simulink model "Hardware_deploy_model"  (R2019a)
settings: Solver=FixedStepDiscrete  StartTime=0.0  StopTime=inf  RelTol=1e-3
model workspace (MAT data in the model file):
  actuatorCentres.aileron.left = 0
  actuatorCentres.aileron.right = 0
  actuatorCentres.elevator.right = 0
  actuatorCentres.elevator.left = 0
  actuatorCentres.flap.left = 0
  actuatorCentres.flap.right = 0
  actuatorCentres.rudder = 0
  loggingSampleTime = Simulink.Parameter
  loggingSampleTime.Value = 1
  loggingSampleTime.DataType = 'double'
  loggingSampleTime.Dimensions = [1 1]
  sensorSampleTime = Simulink.Parameter
  sensorSampleTime.Value = 0.01
  sensorSampleTime.DataType = 'double'
  sensorSampleTime.Dimensions = [1 1]
  servoPins.aileron.left = 9
  servoPins.aileron.right = 10
  servoPins.elevator.left = 7
  servoPins.elevator.right = 8
  servoPins.rudder = 11
  servoPins.flap.left = 5
  servoPins.flap.right = 6
undefined symbols (not defined in the file or in its folder): Aileron, deflectionLimits, DiscIntNeverNeededParam, Discrete, Elevator, Newton, Raphson, Time
libraries: simulink x13, arduinolib x6, ctrlSharedLib x3, aerolibtransform2 x3, sharedtransform x2, aerolibutil x1, simulink_extras x1
settings Model: ExtModeTrigDuration=2  Creator=Aliak  LastModifiedBy=Aliak
settings OptimizationCC: DefaultParameterBehavior=Inlined  GainParamInheritBuiltInType=on  UseFloatMulNetSlope=on  DefaultUnderspecifiedDataType=single  UseSpecifiedMinMax=on  InlineInvariantSignals=on  BitfieldContainerType=uchar_T  MemcpyThreshold=32  PassReuseOutputArgsAs=Individual arguments  ActiveStateOutputEnumStorageType=Smallest  ZeroExternalMemoryAtStartup=off  ZeroInternalMemoryAtStartup=off  NoFixptDivByZeroProtection=on  EfficientFloat2IntCast=on  EfficientMapNaN2IntZero=off  LifeSpan=0.02  MaxStackSize=inf  SimCompilerOptimization=on  OptimizeBlockOrder=speed  DifferentSizesBufferReuse=on
settings DebuggingCC: WriteAfterWriteMsg=EnableAllAsError  AlgebraicLoopMsg=error  IntegerOverflowMsg=error  ParameterUnderflowMsg=error  ParameterPrecisionLossMsg=none  ParameterTunabilityLossMsg=error  AllowSymbolicDim=off  ModelReferenceIOMsg=error  StrictBusMsg=ErrorOnBusTreatedAsVector  NonBusSignalsTreatedAsBus=error  SFInvalidInputDataAccessInChartInitDiag=error  SFTransitionOutsideNaturalParentDiag=error  SFUnreachableExecutionPathDiag=error  SFUndirectedBroadcastEventsDiag=error  SFTransitionActionBeforeConditionDiag=error  IntegerSaturationMsg=error
settings HardwareCC: ProdBitPerInt=16  ProdBitPerPointer=16  ProdBitPerSizeT=16  ProdBitPerPtrDiffT=16  ProdLargestAtomicFloat=None  ProdWordSize=8  ProdLongLongMode=on  ProdHWDeviceType=Atmel->AVR
settings ModelReferenceCC: EnableParallelModelReferenceBuilds=on  ModelReferenceNumInstancesAllowed=Single  ModelReferenceMinAlgLoopOccurrences=on
settings SFSimCC: SimParseCustomCode=off  MATLABDynamicMemAlloc=off
settings RTWCC: SystemTargetFile=ert.tlc  HardwareBoard=Arduino Mega 2560  TemplateMakefile=ert_default_tmf  Toolchain=Arduino AVR  BuildConfiguration=Faster Runs  IncludeHyperlinkInReport=on  CheckMdlBeforeBuild=Warning
settings CodeAppCC: ForceParamTrailComments=on  IgnoreCustomStorageClasses=off  IgnoreTestpoints=on  OperatorAnnotations=on  SimulinkDataObjDesc=on  SFDataObjDesc=on  MATLABFcnDesc=on  InsertBlockDesc=on
settings ERTTargetCC: UtilityFuncGeneration=Shared location  DynamicStringBufferSize=128  IncludeMdlTerminateFcn=off  CombineSignalStateStructs=on  SuppressErrorStatus=on  SupportAbsoluteTime=off  SupportComplex=off  PreserveIfCondition=on
settings ConfigComp: CovScope=ReferencedModels

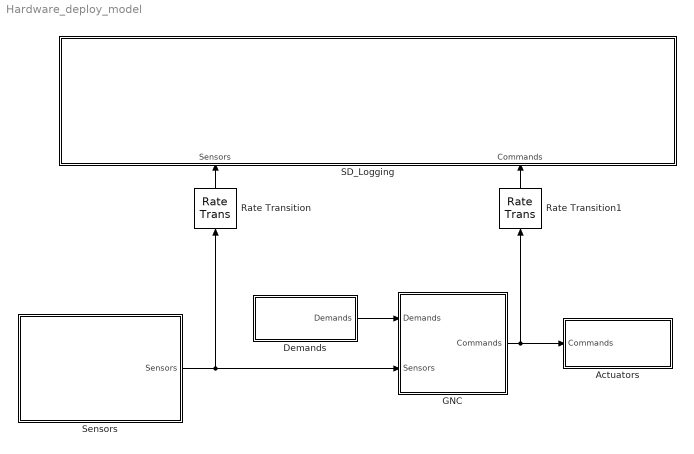
== system Hardware_deploy_model ==
  Actuators : Subsystem  VariantControl=SimType == 1
  Demands : Subsystem
  GNC : Subsystem  VariantControl=SimType==1
  Rate Transition : RateTransition  Deterministic=off  OutPortSampleTime=0.2
  Rate Transition1 : RateTransition  Deterministic=off  OutPortSampleTime=0.2
  SD_Logging : Subsystem  VariantControl=SecArd == 1
  Sensors : Subsystem  VariantControl=SimType==1
  wires:
  Sensors/1(" Sensors") -> GNC/2(Sensors), Rate Transition/1
  GNC/1(Commands) -> Rate Transition1/1, Actuators/1(Commands)
  Rate Transition/1 -> SD_Logging/1("Sensors ")
  Demands/1(Demands) -> GNC/1(Demands)
  Rate Transition1/1 -> SD_Logging/2(Commands)

== system Hardware_deploy_model/Actuators ==
  Commands : Inport  OutDataTypeStr=Bus: Commands
  Aileron Servos : arduinolib/Standard Servo Write  pinNumber=6  ServoIndex=0  blockPlatform=ARDUINO
      settings: SourceProductName=Simulink Support Package for Arduino Hardware
  Bus Selector : BusSelector  OutputSignals=Aileron,Elevator
  Constant : Constant  Value=actuatorCentres.aileron.left  VectorParams1D=off
  Constant1 : Constant  Value=actuatorCentres.elevator.left  VectorParams1D=off
  Elevator Servo : arduinolib/Standard Servo Write  pinNumber=5  ServoIndex=1  blockPlatform=ARDUINO
      settings: SourceProductName=Simulink Support Package for Arduino Hardware
  Initialize Function : Subsystem  Commented=on  TreatAsAtomicUnit=on
  Saturation : Saturate  Commented=through  UpperLimit=deflectionLimits.aileron.max  LowerLimit=deflectionLimits.aileron.min
  Saturation1 : Saturate  Commented=through  UpperLimit=deflectionLimits.elevator.max  LowerLimit=deflectionLimits.elevator.min
  Subtract : Sum  Inputs=-+  RndMeth=Simplest
  Subtract1 : Sum  Inputs=-+
  wires:
  Commands/1 -> Bus Selector/1
  Saturation1/1 -> Subtract1/2
  Bus Selector/2 -> Saturation1/1  "<Elevator>"
  Subtract1/1 -> Elevator Servo/1
  Constant1/1 -> Subtract1/1
  Bus Selector/1 -> Saturation/1  "<Aileron>"
  Saturation/1 -> Subtract/2
  Constant/1 -> Subtract/1
  Subtract/1 -> Aileron Servos/1

== system Hardware_deploy_model/Demands ==
  Bus Creator : BusCreator  Inputs=2  OutDataTypeStr=Bus: Demands
  Constant : Constant  Value=90  VectorParams1D=off  OutDataTypeStr=single
  Constant1 : Constant  Value=60  VectorParams1D=off  OutDataTypeStr=single
  Demands : Outport
  wires:
  Constant/1 -> Bus Creator/1  "Heading"
  Constant1/1 -> Bus Creator/2  "Altitude"
  Bus Creator/1 -> Demands/1

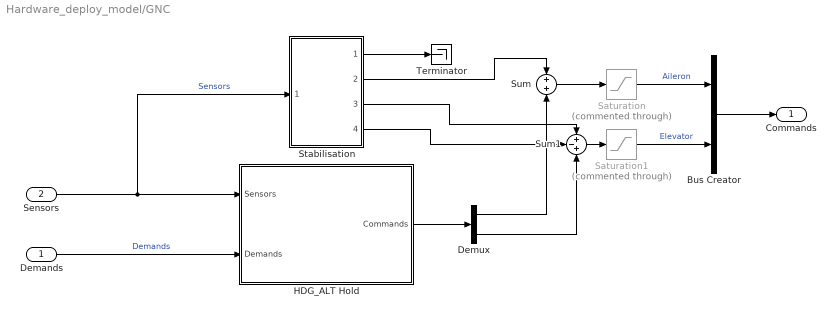
== system Hardware_deploy_model/GNC ==
  Demands : Inport  OutDataTypeStr=Bus: Demands
  Sensors : Inport  Port=2  OutDataTypeStr=Bus: Sensors
  Bus Creator : BusCreator  Inputs=Aileron,Elevator  OutDataTypeStr=Bus: Commands
  Demux : Demux  Outputs=2
  HDG_ALT Hold : Subsystem
  Saturation : Saturate  Commented=through  UpperLimit=deflectionLimits.aileron.max  LowerLimit=deflectionLimits.aileron.min
  Saturation1 : Saturate  Commented=through  UpperLimit=deflectionLimits.elevator.max  LowerLimit=deflectionLimits.elevator.min
  Stabilisation : Subsystem
  Sum : Sum
  Sum1 : Sum  Inputs=+-+
  Terminator : Terminator
  Commands : Outport
  wires:
  Bus Creator/1 -> Commands/1
  Sum/1 -> Saturation/1
  Sum1/1 -> Saturation1/1
  HDG_ALT Hold/1(Commands) -> Demux/1
  Demux/1 -> Sum/2
  Sensors/1 -> Stabilisation/1(Sensors), HDG_ALT Hold/1(Sensors)  "Sensors"
  Demands/1 -> HDG_ALT Hold/2(Demands)  "Demands"
  Demux/2 -> Sum1/3
  Stabilisation/2(Roll Stab) -> Sum/1
  Stabilisation/3(Pitch Stab) -> Sum1/1
  Stabilisation/1(Yaw Stab) -> Terminator/1
  Stabilisation/4(Stall Stab) -> Sum1/2
  Saturation/1 -> Bus Creator/1  "Aileron"
  Saturation1/1 -> Bus Creator/2  "Elevator"

== system Hardware_deploy_model/SD_Logging ==
  "Sensors " : Inport  OutDataTypeStr=Bus: Sensors
  Commands : Inport  Port=2  OutDataTypeStr=Bus: Commands
  Bus Selector : BusSelector  OutputSignals=X_e,V_e,phi_theta_psi,pqr
  Bus Selector1 : BusSelector  OutputSignals=Aileron,Elevator
  Demux{,1..3} (4 alike) : Demux  Outputs=3
  MATLAB System : MATLABSystem  System=SDLogger  SimulateUsing=Code generation
      mask Type: SDLogger
      mask Display:
      | disp('SDLogger');
      | port_label('input',1,'data');
  Mux : Mux  Inputs=14
  wires:
  "Sensors "/1 -> Bus Selector/1
  Bus Selector/1 -> Demux/1  "<X_e>"
  Bus Selector/3 -> Demux1/1  "<phi_theta_psi>"
  Bus Selector/4 -> Demux2/1  "<pqr>"
  Bus Selector/2 -> Demux3/1  "<V_e>"
  Demux/1 -> Mux/1
  Demux/2 -> Mux/2
  Demux/3 -> Mux/3
  Demux3/1 -> Mux/4
  Demux3/2 -> Mux/5
  Demux3/3 -> Mux/6
  Demux1/1 -> Mux/7
  Demux1/2 -> Mux/8
  Demux1/3 -> Mux/9
  Demux2/1 -> Mux/10
  Demux2/2 -> Mux/11
  Demux2/3 -> Mux/12
  Mux/1 -> MATLAB System/1
  Commands/1 -> Bus Selector1/1
  Bus Selector1/1 -> Mux/13  "<Aileron>"
  Bus Selector1/2 -> Mux/14  "<Elevator>"

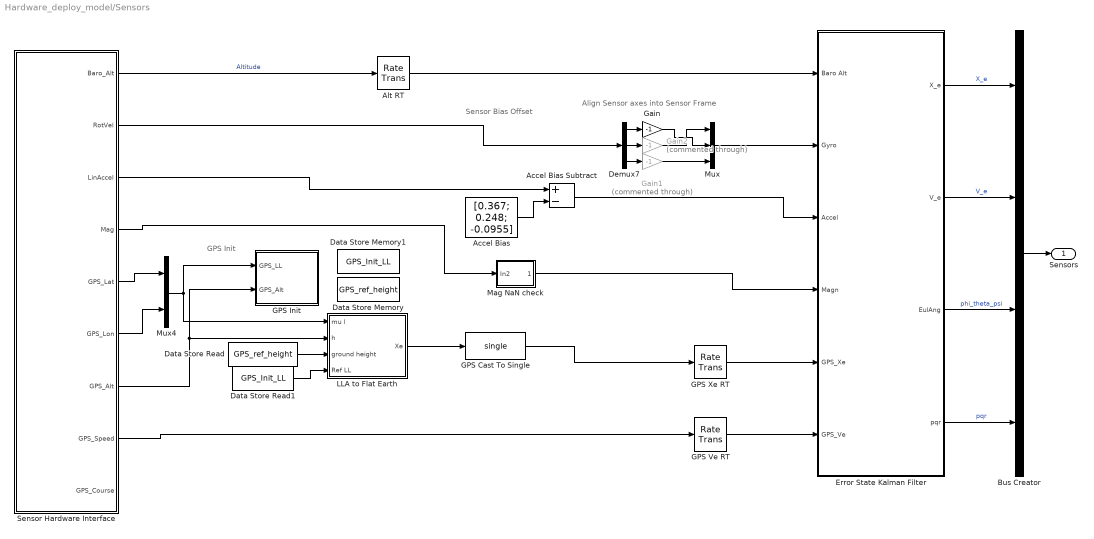
== system Hardware_deploy_model/Sensors ==
  note: GPS Init
  note: Sensor Bias Offset
  note: Align Sensor axes into Sensor Frame
  Accel Bias : Constant  Value=[0.367; 0.248; -0.0955]  VectorParams1D=off
  Accel Bias Subtract : Sum  Inputs=+-  OutDataTypeStr=single
  Alt RT : RateTransition  Deterministic=off
  Bus Creator : BusCreator  Inputs=4  OutDataTypeStr=Bus: Sensors
      settings: InheritFromInputs=off
  Data Store Memory : DataStoreMemory  DataStoreName=GPS_ref_height  ReadBeforeWriteMsg=warning  WriteAfterWriteMsg=warning  WriteAfterReadMsg=warning  ShowAdditionalParam=off  OutDataTypeStr=single
  Data Store Memory1 : DataStoreMemory  DataStoreName=GPS_Init_LL  ReadBeforeWriteMsg=warning  WriteAfterWriteMsg=warning  WriteAfterReadMsg=warning  InitialValue=[0 0]  ShowAdditionalParam=off  OutDataTypeStr=single
  Data Store Read : DataStoreRead  DataStoreName=GPS_ref_height  DataStoreElements=GPS_ref_height
  Data Store Read1 : DataStoreRead  DataStoreName=GPS_Init_LL
  Demux7 : Demux  Outputs=3
  Error State Kalman Filter : Subsystem
  GPS Cast To Single : DataTypeConversion  OutDataTypeStr=single  RndMeth=Simplest
  GPS Init : Subsystem
  GPS Ve RT : RateTransition  Deterministic=off
  GPS Xe RT : RateTransition  Deterministic=off
  Gain : Gain  Gain=-1
  Gain1 : Gain  Commented=through  Gain=-1
  Gain2 : Gain  Commented=through  Gain=-1
  LLA to Flat Earth : Subsystem
  Mag NaN check : Subsystem
  Mux : Mux  Inputs=3
  Mux4 : Mux  Inputs=2
  Sensor Hardware Interface : Subsystem  VariantControl=SimType==1
  " Sensors" : Outport
  wires:
  Error State Kalman Filter/3(EulAng) -> Bus Creator/3  "phi_theta_psi"
  Error State Kalman Filter/2(V_e) -> Bus Creator/2  "V_e"
  Error State Kalman Filter/1(X_e) -> Bus Creator/1  "X_e"
  Error State Kalman Filter/4(pqr) -> Bus Creator/4  "pqr"
  Bus Creator/1 -> " Sensors"/1
  GPS Ve RT/1 -> Error State Kalman Filter/6(GPS_Ve)
  GPS Cast To Single/1 -> GPS Xe RT/1
  Sensor Hardware Interface/1(Baro_Alt) -> Alt RT/1  "Altitude"
  Sensor Hardware Interface/4(Mag) -> Mag NaN check/1(In2)
  Demux7/3 -> Gain1/1
  Sensor Hardware Interface/7(GPS_Alt) -> LLA to Flat Earth/2(h), GPS Init/2(GPS_Alt)
  Sensor Hardware Interface/5(GPS_Lat) -> Mux4/1
  Data Store Read1/1 -> LLA to Flat Earth/4(Ref LL)
  Sensor Hardware Interface/8(GPS_Speed) -> GPS Ve RT/1
  Sensor Hardware Interface/6(GPS_Lon) -> Mux4/2
  LLA to Flat Earth/1(Xe) -> GPS Cast To Single/1
  Gain1/1 -> Mux/3
  Demux7/1 -> Gain/1
  Mag NaN check/1(Out1) -> Error State Kalman Filter/4(Magn)
  Accel Bias Subtract/1 -> Error State Kalman Filter/3(Accel)
  Mux/1 -> Error State Kalman Filter/2(Gyro)
  Sensor Hardware Interface/2(RotVel) -> Demux7/1
  Alt RT/1 -> Error State Kalman Filter/1(Baro Alt)
  Gain/1 -> Mux/2
  Sensor Hardware Interface/3(LinAccel) -> Accel Bias Subtract/1
  Data Store Read/1 -> LLA to Flat Earth/3(ground height)
  GPS Xe RT/1 -> Error State Kalman Filter/5(GPS_Xe)
  Mux4/1 -> LLA to Flat Earth/1(mu l), GPS Init/1(GPS_LL)
  Gain2/1 -> Mux/1
  Accel Bias/1 -> Accel Bias Subtract/2
  Demux7/2 -> Gain2/1

== system Hardware_deploy_model/Actuators/Initialize Function ==
  Aileron Servos : arduinolib/Standard Servo Write  pinNumber=servoPins.aileron.right  ServoIndex=0  blockPlatform=ARDUINO
      settings: SourceProductName=Simulink Support Package for Arduino Hardware
  Elevator Servo : arduinolib/Standard Servo Write  pinNumber=servoPins.elevator.right  ServoIndex=0  blockPlatform=ARDUINO
      settings: SourceProductName=Simulink Support Package for Arduino Hardware
  Event Listener : EventListener  DisableCoverage=on  EventName=reset
  Flap Servo : arduinolib/Standard Servo Write  pinNumber=servoPins.flap.right  ServoIndex=0  blockPlatform=ARDUINO
      settings: SourceProductName=Simulink Support Package for Arduino Hardware
  Rudder Servo : arduinolib/Standard Servo Write  pinNumber=servoPins.rudder  ServoIndex=0  blockPlatform=ARDUINO
      settings: SourceProductName=Simulink Support Package for Arduino Hardware
  Step : Step  After=180  SampleTime=0
  Step1 : Step  Time=6  After=180  SampleTime=0
  Sum : Sum  Inputs=+-
  wires:
  Sum/1 -> Flap Servo/1, Rudder Servo/1, Elevator Servo/1, Aileron Servos/1
  Step/1 -> Sum/1
  Step1/1 -> Sum/2

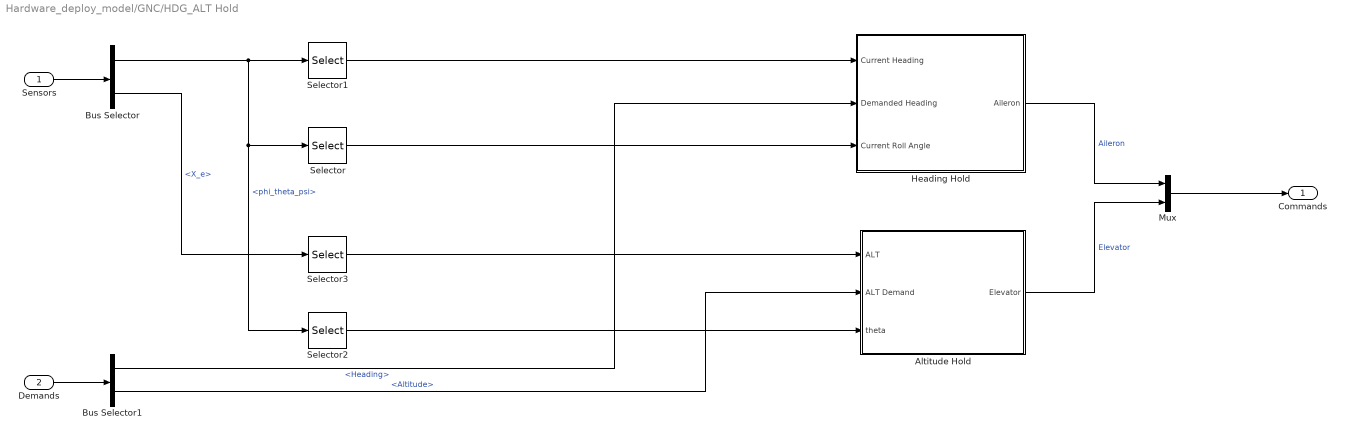
== system Hardware_deploy_model/GNC/HDG_ALT Hold ==
  Sensors : Inport  OutDataTypeStr=Bus: Sensors
  Demands : Inport  Port=2  OutDataTypeStr=Bus: Demands
  Altitude Hold : Subsystem
      settings: UndoDeleteFcn=Stateflow.SLINSF.SimulinkMan.restorePreDeleteFcn  PreDeleteFcn=Stateflow.SLINSF.SimulinkMan.removePreDeleteFcn
  Bus Selector : BusSelector  OutputSignals=phi_theta_psi,X_e
  Bus Selector1 : BusSelector  OutputSignals=Heading,Altitude
  Heading Hold : Subsystem
  Mux : Mux  Inputs=2
  Selector : Selector  IndexMode=Zero-based  InputPortWidth=3  IndexOptions=Index vector (dialog)  Indices=[0]  OutputSizes=1
  Selector1 : Selector  IndexMode=Zero-based  InputPortWidth=3  IndexOptions=Index vector (dialog)  Indices=[2]  OutputSizes=1
  Selector2 : Selector  IndexMode=Zero-based  InputPortWidth=3  IndexOptions=Index vector (dialog)  Indices=[1]  OutputSizes=1
  Selector3 : Selector  IndexMode=Zero-based  InputPortWidth=3  IndexOptions=Index vector (dialog)  Indices=[2]  OutputSizes=1
  Commands : Outport
  wires:
  Selector1/1 -> Heading Hold/1(Current Heading)
  Selector3/1 -> Altitude Hold/1(ALT)
  Bus Selector1/2 -> Altitude Hold/2(ALT Demand)  "<Altitude>"
  Bus Selector/1 -> Selector1/1, Selector/1, Selector2/1  "<phi_theta_psi>"
  Bus Selector1/1 -> Heading Hold/2(Demanded Heading)  "<Heading>"
  Bus Selector/2 -> Selector3/1  "<X_e>"
  Demands/1 -> Bus Selector1/1
  Selector/1 -> Heading Hold/3(Current Roll Angle)
  Sensors/1 -> Bus Selector/1
  Selector2/1 -> Altitude Hold/3(theta)
  Altitude Hold/1(Elevator) -> Mux/2  "Elevator"
  Mux/1 -> Commands/1
  Heading Hold/1(Aileron) -> Mux/1  "Aileron"

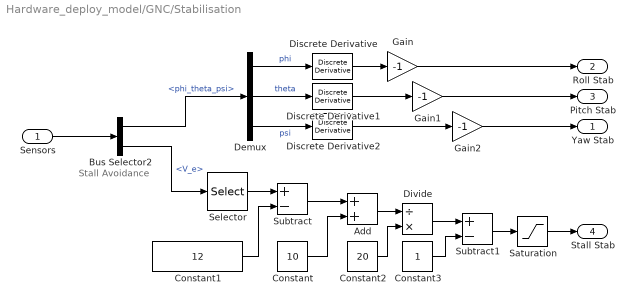
== system Hardware_deploy_model/GNC/Stabilisation ==
  note: Stall Avoidance
  Sensors : Inport
  Add : Sum
  Bus Selector2 : BusSelector  OutputSignals=phi_theta_psi,V_e
  Constant : Constant  Value=10  OutDataTypeStr=single
  Constant1 : Constant  Value=12  OutDataTypeStr=single
  Constant2 : Constant  Value=20  OutDataTypeStr=single
  Constant3 : Constant  OutDataTypeStr=single
  Demux : Demux  Outputs=3
  Discrete Derivative : simulink/Discrete/Discrete Derivative  gainval=1.0  ICPrevScaledInput=0.0  OutMin=-50  OutMax=50  OutDataType=fixdt(1, 16)  OutScaling=2^-10  RndMeth=Simplest  DoSatur=on
  Discrete Derivative1 : simulink/Discrete/Discrete Derivative  gainval=1.0  ICPrevScaledInput=0.0  OutMin=-50  OutMax=50  OutDataType=fixdt(1, 16)  OutScaling=2^-10  RndMeth=Simplest  DoSatur=on
  Discrete Derivative2 : simulink/Discrete/Discrete Derivative  gainval=1.0  ICPrevScaledInput=0.0  OutMin=-50  OutMax=50  OutDataType=fixdt(1, 16)  OutScaling=2^-10  RndMeth=Simplest  DoSatur=on
  Divide : Product  Inputs=/*
  Gain : Gain  Gain=-1
  Gain1 : Gain  Gain=-1
  Gain2 : Gain  Gain=-1
  Saturation : Saturate  UpperLimit=1  LowerLimit=0
  Selector : Selector  IndexMode=Zero-based  InputPortWidth=3  IndexOptions=Index vector (dialog)  Indices=[0]  OutputSizes=1
  Subtract : Sum  Inputs=+-
  Subtract1 : Sum  Inputs=+-
  Yaw Stab : Outport
  Roll Stab : Outport  Port=2
  Pitch Stab : Outport  Port=3
  Stall Stab : Outport  Port=4
  wires:
  Gain2/1 -> Yaw Stab/1
  Bus Selector2/2 -> Selector/1  "<V_e>"
  Discrete Derivative2/1 -> Gain2/1
  Selector/1 -> Subtract/1
  Sensors/1 -> Bus Selector2/1
  Demux/2 -> Discrete Derivative1/1  "theta"
  Demux/1 -> Discrete Derivative/1  "phi"
  Demux/3 -> Discrete Derivative2/1  "psi"
  Discrete Derivative1/1 -> Gain1/1
  Discrete Derivative/1 -> Gain/1
  Bus Selector2/1 -> Demux/1  "<phi_theta_psi>"
  Gain/1 -> Roll Stab/1
  Gain1/1 -> Pitch Stab/1
  Constant1/1 -> Subtract/2
  Saturation/1 -> Stall Stab/1
  Subtract/1 -> Add/1
  Constant/1 -> Add/2
  Add/1 -> Divide/1
  Constant2/1 -> Divide/2
  Divide/1 -> Subtract1/1
  Constant3/1 -> Subtract1/2
  Subtract1/1 -> Saturation/1

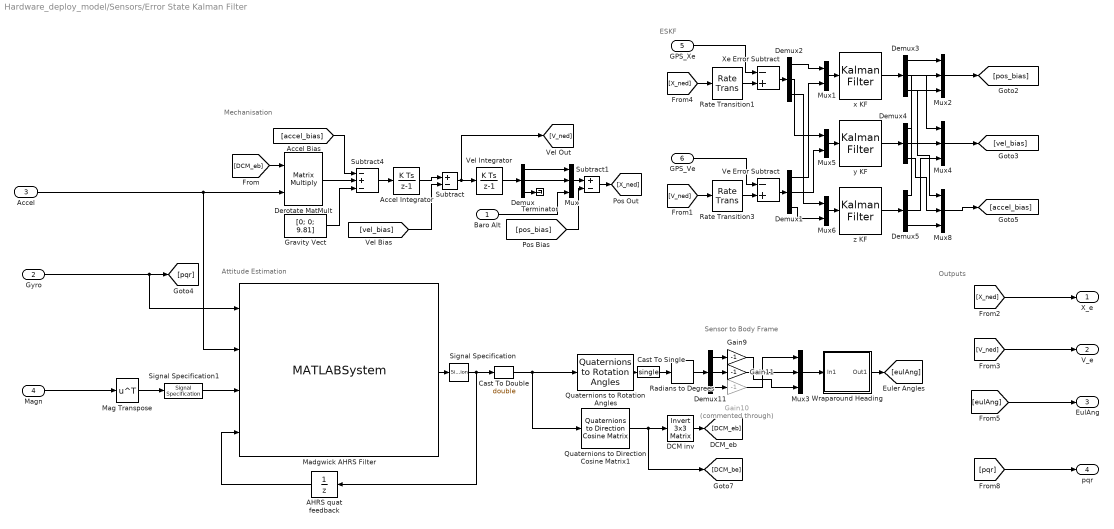
== system Hardware_deploy_model/Sensors/Error State Kalman Filter ==
  note: Attitude Estimation
  note: Mechanisation
  note: ESKF
  note: Outputs
  note: Sensor to Body Frame
  Baro Alt : Inport
  Gyro : Inport  Port=2
  Accel : Inport  Port=3
  Magn : Inport  Port=4
  GPS_Xe : Inport  Port=5
  GPS_Ve : Inport  Port=6
  AHRS quat feedback : UnitDelay  InitialCondition=[1 0 0 0]  SampleTime=sensorSampleTime  HasFrameUpgradeWarning=on
  Accel Integrator : DiscreteIntegrator  gainval=1  SampleTime=-1  ICPrevOutput=DiscIntNeverNeededParam  ICPrevScaledInput=DiscIntNeverNeededParam
  Cast To Double : DataTypeConversion  OutDataTypeStr=double
  Cast To Single : DataTypeConversion  OutDataTypeStr=single
  DCM inv : aerolibutil/Invert  3x3 Matrix
  Demux{,1..5,11} (7 alike) : Demux  Outputs=3
  Derotate MatMult : Product  Multiplication=Matrix(*)  OutDataTypeStr=single  RndMeth=Simplest
  Gain10 : Gain  Commented=through  Gain=-1
  Gain11 : Gain  Gain=-1
  Gain9 : Gain  Gain=-1
  Gravity Vect : Constant  Value=[0; 0; 9.81]  VectorParams1D=off  OutDataTypeStr=single
  Madgwick AHRS Filter : MATLABSystem  System=MadgwickAHRSFilter  SamplePeriod=sensorSampleTime  Beta=1  SimulateUsing=Code generation
      mask Type: MadgwickAHRSFilter
      mask Display:
      | disp('MadgwickAHRSFilter');
      | port_label('input',1,'Gyroscope');
      | port_label('input',2,'Accelerometer');
      | port_label('input',3,'Magnetometer');
      | port_label('input',4,'q');
      | port_label('output',1,'quat');
  Mag Transpose : Math  Operator=transpose  SaturateOnIntegerOverflow=on
  Mux{,2..4,8} (5 alike) : Mux  Inputs=3
  Mux1 : Mux  Inputs=2
  Mux5 : Mux  Inputs=2
  Mux6 : Mux  Inputs=2
  Quaternions to Direction Cosine Matrix1 : sharedtransform/Quaternions to  Direction Cosine Matrix  aMode=aMode
      settings: SourceProductName=Aerospace Blockset  SourceProductBaseCode=AE
  Quaternions to Rotation Angles : sharedtransform/Quaternions to Rotation Angles  rotationOrder=ZYX  aMode=aMode
      settings: SourceProductBaseCode=AE
  Radians to Degrees : simulink_extras/Transformations/Radians to Degrees
  Rate Transition1 : RateTransition  Deterministic=off  OutPortSampleTime=1
  Rate Transition3 : RateTransition  Deterministic=off  OutPortSampleTime=1
  Signal Specification : SignalSpecification  OutDataTypeStr=single  Dimensions=[1 4]
  Signal Specification1 : SignalSpecification  OutDataTypeStr=single  Dimensions=[1 3]
  Subtract : Sum  Inputs=+-
  Subtract1 : Sum  Inputs=+-
  Subtract4 : Sum  Inputs=-+-  AccumDataTypeStr=single
  Terminator : Terminator
  Ve Error Subtract : Sum  Inputs=-+  AccumDataTypeStr=single  OutDataTypeStr=single  RndMeth=Simplest
  Vel Integrator : DiscreteIntegrator  gainval=1  SampleTime=-1  OutDataTypeStr=single  ICPrevOutput=DiscIntNeverNeededParam  ICPrevScaledInput=DiscIntNeverNeededParam
  Wraparound Heading : Subsystem
  Xe Error Subtract : Sum  Inputs=-+  AccumDataTypeStr=single  OutDataTypeStr=single  RndMeth=Simplest
  x KF : ctrlSharedLib/Kalman Filter  TimeDomain=Discrete-Time  UseCurrentEstimator=off  ModelSource=Individual A, B, C, D matrices  ModelSourceVariable=ss(0.95,1,1,0,1)  A=[1 0.2 0.02; 0 1 0.2; 0 0 1]  B=0  C=[1 0 0; 0 1 0]  D=0  NumberOfStates=3  NumberOfInputs=1  NumberOfOutputs=3  InitialEstimateSource=Dialog  X0=[0;0;0]  P0=10  UseK=off  UseGH=off  NumberOfProcessNoiseInputs=1  G=1  TimeInvariantG=on  H=0  TimeInvariantH=on  Q=1  TimeInvariantQ=on  R=0.1  TimeInvariantR=on  N=0  TimeInvariantN=on  AddInputPort=off  AddEnablePort=off  OutputEstimatedY=off  OutputP=off  Ts=1
      settings: SourceProductBaseCode=CT
  y KF : ctrlSharedLib/Kalman Filter  TimeDomain=Discrete-Time  UseCurrentEstimator=off  ModelSource=Individual A, B, C, D matrices  ModelSourceVariable=ss(0.95,1,1,0,1)  A=[1 1 0.5; 0 1 1; 0 0 1]  B=0  C=[1 0 0; 0 1 0]  D=0  NumberOfStates=3  NumberOfInputs=1  NumberOfOutputs=3  InitialEstimateSource=Dialog  X0=[0;0;0]  P0=10  UseK=off  UseGH=off  NumberOfProcessNoiseInputs=1  G=1  TimeInvariantG=on  H=0  TimeInvariantH=on  Q=1  TimeInvariantQ=on  R=0.1  TimeInvariantR=on  N=0  TimeInvariantN=on  AddInputPort=off  AddEnablePort=off  OutputEstimatedY=off  OutputP=off  Ts=1
      settings: SourceProductBaseCode=CT
  z KF : ctrlSharedLib/Kalman Filter  TimeDomain=Discrete-Time  UseCurrentEstimator=off  ModelSource=Individual A, B, C, D matrices  ModelSourceVariable=ss(0.95,1,1,0,1)  A=[1 1 0.5; 0 1 1; 0 0 1]  B=0  C=[1 0 0; 0 1 0]  D=0  NumberOfStates=3  NumberOfInputs=1  NumberOfOutputs=3  InitialEstimateSource=Dialog  X0=[0;0;0]  P0=10  UseK=off  UseGH=off  NumberOfProcessNoiseInputs=1  G=1  TimeInvariantG=on  H=0  TimeInvariantH=on  Q=1  TimeInvariantQ=on  R=0.1  TimeInvariantR=on  N=0  TimeInvariantN=on  AddInputPort=off  AddEnablePort=off  OutputEstimatedY=off  OutputP=off  Ts=1
      settings: SourceProductBaseCode=CT
  X_e : Outport
  V_e : Outport  Port=2
  EulAng : Outport  Port=3
  pqr : Outport  Port=4
  wires:
  Accel/1 -> Madgwick AHRS Filter/2, Derotate MatMult/2
  [DCM_eb] -> Derotate MatMult/1
  Derotate MatMult/1 -> Subtract4/2
  Vel Integrator/1 -> Demux/1
  Demux/1 -> Mux/1
  Demux/2 -> Mux/2
  Baro Alt/1 -> Mux/3
  Demux/3 -> Terminator/1
  GPS_Xe/1 -> Xe Error Subtract/1
  GPS_Ve/1 -> Ve Error Subtract/1
  Subtract4/1 -> Accel Integrator/1
  Gravity Vect/1 -> Subtract4/3
  Mux/1 -> Subtract1/1
  Accel Integrator/1 -> Subtract/1
  [X_ned] -> X_e/1
  [V_ned] -> V_e/1
  AHRS quat feedback/1 -> Madgwick AHRS Filter/4
  Demux11/3 -> Gain10/1
  Quaternions to Rotation Angles/1 -> Cast To Single/1
  Gain9/1 -> Mux3/3
  Gain11/1 -> Mux3/2
  Demux11/1 -> Gain9/1
  Wraparound Heading/1(Out1) -> [eulAng]
  Madgwick AHRS Filter/1 -> Signal Specification/1
  Gain10/1 -> Mux3/1
  Demux11/2 -> Gain11/1
  Radians to Degrees/1 -> Demux11/1
  Mux3/1 -> Wraparound Heading/1(In1)
  DCM inv/1 -> [DCM_eb]
  Quaternions to Direction Cosine Matrix1/1 -> [DCM_be], DCM inv/1
  Gyro/1 -> Madgwick AHRS Filter/1, [pqr]
  Mag Transpose/1 -> Signal Specification1/1
  [pqr] -> pqr/1
  Magn/1 -> Mag Transpose/1
  [eulAng] -> EulAng/1
  Signal Specification1/1 -> Madgwick AHRS Filter/3
  Subtract/1 -> Vel Integrator/1, [V_ned]
  [V_ned] -> Rate Transition3/1
  [X_ned] -> Rate Transition1/1
  Mux1/1 -> x KF/1
  Mux5/1 -> y KF/1
  Mux6/1 -> z KF/1
  Demux2/1 -> Mux1/1
  Demux1/1 -> Mux1/2
  Demux2/2 -> Mux5/1
  Demux1/2 -> Mux5/2
  Demux2/3 -> Mux6/1
  Demux1/3 -> Mux6/2
  x KF/1 -> Demux3/1
  y KF/1 -> Demux4/1
  z KF/1 -> Demux5/1
  Demux3/1 -> Mux2/1
  Demux4/1 -> Mux2/2
  Demux5/1 -> Mux2/3
  Demux3/2 -> Mux4/1
  Demux4/2 -> Mux4/2
  Demux5/2 -> Mux4/3
  Demux3/3 -> Mux8/1
  Demux4/3 -> Mux8/2
  Demux5/3 -> Mux8/3
  [accel_bias] -> Subtract4/1
  [vel_bias] -> Subtract/2
  Subtract1/1 -> [X_ned]
  [pos_bias] -> Subtract1/2
  Xe Error Subtract/1 -> Demux2/1
  Ve Error Subtract/1 -> Demux1/1
  Rate Transition1/1 -> Xe Error Subtract/2
  Rate Transition3/1 -> Ve Error Subtract/2
  Cast To Single/1 -> Radians to Degrees/1
  Signal Specification/1 -> Cast To Double/1, AHRS quat feedback/1
  Mux2/1 -> [pos_bias]
  Mux4/1 -> [vel_bias]
  Mux8/1 -> [accel_bias]
  Cast To Double/1 -> Quaternions to Rotation Angles/1, Quaternions to Direction Cosine Matrix1/1

== system Hardware_deploy_model/Sensors/GPS Init ==
  GPS_LL : Inport
  GPS_Alt : Inport  Port=2
  Constant : Constant  Value=0  OutDataTypeStr=single
  Data Store Memory : DataStoreMemory  DataStoreName=GPS_init  ReadBeforeWriteMsg=warning  WriteAfterWriteMsg=warning  WriteAfterReadMsg=warning  InitialValue=true  ShowAdditionalParam=off  OutDataTypeStr=boolean
  Data Store Read : DataStoreRead  DataStoreName=GPS_init  DataStoreElements=GPS_init
  Equal : RelationalOperator  Operator=~=  OutDataTypeStr=boolean  RndMeth=Simplest
  If : If  NumInputs=2  IfExpression=u1 & u2  ShowElse=off
  If Action Subsystem : Subsystem  TreatAsAtomicUnit=on
  wires:
  Data Store Read/1 -> If/1
  If/1 -> If Action Subsystem/Action
  GPS_Alt/1 -> Equal/2, If Action Subsystem/2(GPS_Alt)
  GPS_LL/1 -> If Action Subsystem/1(GPS_LL)
  Equal/1 -> If/2
  Constant/1 -> Equal/1

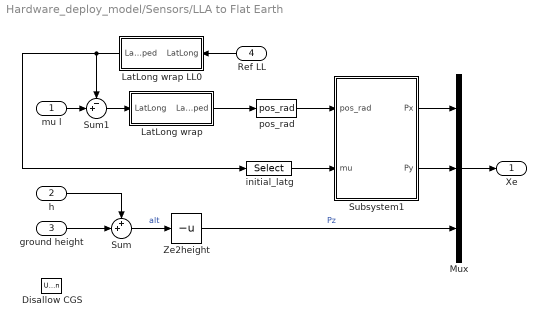
== system Hardware_deploy_model/Sensors/LLA to Flat Earth ==
  mu l : Inport  Unit=deg
  h : Inport  Port=2  Unit=m
  ground height : Inport  Port=3  Unit=m
  Ref LL : Inport  Port=4
  Disallow CGS : UnitConfiguration  UnitSystemsStr=English,SI,SI (extended)  AllowAllUnitSystems=off
  LatLong wrap : Subsystem  AncestorBlock=aerolibtransform2sys/LatLong wrap
      mask init:
      | aeroicon('aeroblk')
      mask Display:
      | port_label('input',1,'[\mu l]','texmode','on')
      | port_label('output',1,'[\mu l]_{wrap}','texmode','on')
  LatLong wrap LL0 : Subsystem  AncestorBlock=aerolibtransform2sys/LatLong wrap
      mask init:
      | aeroicon('aeroblk')
      mask Display:
      | port_label('input',1,'[\mu l]','texmode','on')
      | port_label('output',1,'[\mu l]_{wrap}','texmode','on')
  Mux : Mux  Inputs=3
  Subsystem1 : Subsystem
  Sum : Sum  Inputs=++|
  Sum1 : Sum  Inputs=-+|
  Ze2height : UnaryMinus
  initial_latg : Selector  IndexMode=Zero-based  InputPortWidth=2  IndexOptions=Index vector (dialog)  Indices=[1]  OutputSizes=1
  pos_rad : aerolibtransform2/LLA to Flat Earth/pos_rad  SystemSampleTime=-1
      settings: SourceProductName=Aerospace Blockset  SourceProductBaseCode=AE
  Xe : Outport  Unit=m
  wires:
  LatLong wrap LL0/1(Lat/Long wrapped) -> initial_latg/1, Sum1/1
  pos_rad/1 -> Subsystem1/1(pos_rad)
  Sum1/1 -> LatLong wrap/1(LatLong)
  Subsystem1/2(Py) -> Mux/2
  Subsystem1/1(Px) -> Mux/1
  Ze2height/1 -> Mux/3  "Pz"
  Mux/1 -> Xe/1
  initial_latg/1 -> Subsystem1/2(mu)
  h/1 -> Sum/1
  Ref LL/1 -> LatLong wrap LL0/1(LatLong)
  ground height/1 -> Sum/2
  mu l/1 -> Sum1/2
  LatLong wrap/1(Lat/Long wrapped) -> pos_rad/1
  Sum/1 -> Ze2height/1  "alt"

== system Hardware_deploy_model/Sensors/Mag NaN check ==
  In2 : Inport
  Relational Operator1 : RelationalOperator  Operator=isNaN  OutDataTypeStr=boolean  RndMeth=Simplest
  Switch1 : Switch  Criteria=u2 ~= 0
  Unit Delay5 : UnitDelay  InitialCondition=[0; 0; 0]  SampleTime=-1  HasFrameUpgradeWarning=on
  Out1 : Outport
  wires:
  Relational Operator1/1 -> Switch1/2
  Unit Delay5/1 -> Switch1/1
  Switch1/1 -> Unit Delay5/1, Out1/1
  In2/1 -> Relational Operator1/1, Switch1/3

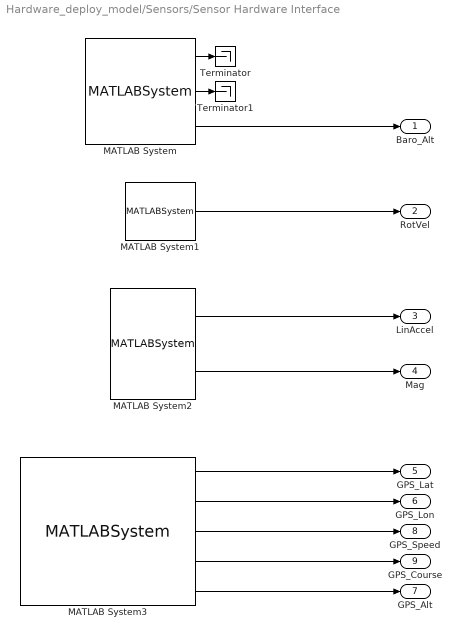
== system Hardware_deploy_model/Sensors/Sensor Hardware Interface ==
  MATLAB System : MATLABSystem  System=BMP085  Reference_Pressure=101200  SimulateUsing=Code generation
      mask Type: BMP085
      mask Display:
      | disp('BMP085');
      | port_label('output',1,'press');
      | port_label('output',2,'temp');
      | port_label('output',3,'alt');
  MATLAB System1 : MATLABSystem  System=L3GD20  SimulateUsing=Code generation
      mask Type: L3GD20
      mask Display:
      | disp('L3GD20');
      | port_label('output',1,'rot');
  MATLAB System2 : MATLABSystem  System=LSM303  SimulateUsing=Code generation
      mask Type: LSM303
      mask Display:
      | disp('LSM303');
      | port_label('output',1,'accel');
      | port_label('output',2,'mag');
  MATLAB System3 : MATLABSystem  System=TinyGPS  SimulateUsing=Code generation
      mask Type: TinyGPS
      mask Display:
      | disp('TinyGPS');
      | port_label('output',1,'lat');
      | port_label('output',2,'lon');
      | port_label('output',3,'speed');
      | port_label('output',4,'course');
      | port_label('output',5,'alt');
  Terminator : Terminator
  Terminator1 : Terminator
  Baro_Alt : Outport
  RotVel : Outport  Port=2
  LinAccel : Outport  Port=3
  Mag : Outport  Port=4
  GPS_Lat : Outport  Port=5
  GPS_Lon : Outport  Port=6
  GPS_Alt : Outport  Port=7
  GPS_Speed : Outport  Port=8
  GPS_Course : Outport  Port=9
  wires:
  MATLAB System/3 -> Baro_Alt/1
  MATLAB System1/1 -> RotVel/1
  MATLAB System2/1 -> LinAccel/1
  MATLAB System2/2 -> Mag/1
  MATLAB System/1 -> Terminator/1
  MATLAB System/2 -> Terminator1/1
  MATLAB System3/1 -> GPS_Lat/1
  MATLAB System3/2 -> GPS_Lon/1
  MATLAB System3/3 -> GPS_Speed/1
  MATLAB System3/5 -> GPS_Alt/1
  MATLAB System3/4 -> GPS_Course/1

== system Hardware_deploy_model/GNC/HDG_ALT Hold/Altitude Hold ==
  ALT : Inport
  ALT Demand : Inport  Port=2
  theta : Inport  Port=3
  Altitude Hold : Subsystem
  Elevator : Outport
  wires:
  Altitude Hold/1(Elevator) -> Elevator/1
  ALT/1 -> Altitude Hold/1(In1)
  ALT Demand/1 -> Altitude Hold/2(In2)
  theta/1 -> Altitude Hold/3(theta)

== system Hardware_deploy_model/GNC/HDG_ALT Hold/Heading Hold ==
  Current Heading : Inport
  Demanded Heading : Inport  Port=2
  Current Roll Angle : Inport  Port=3
  Aileron Controller : simulink/Continuous/PID Controller  Controller=PID  Form=Parallel  TimeDomain=Discrete-time  SampleTime=-1  IntegratorMethod=Forward Euler  FilterMethod=Forward Euler  ControllerParametersSource=internal  P=1  I=1  D=0  UseFilter=on  N=100  TunerSelectOption=Transfer Function Based (PID Tuner App)  InitialConditionSource=internal  InitialConditionForIntegrator=0  InitialConditionForFilter=0  DifferentiatorICPrevScaledInput=0  ExternalReset=none  TrackingMode=off  Kt=1  LimitOutput=on  UpperSaturationLimit=500  LowerSaturationLimit=-500  LinearizeAsGain=off  AntiWindupMode=none  Kb=1  RndMeth=Simplest  POutMin=[]  POutMax=[]  IOutMin=[]  IOutMax=[]  DOutMin=[]  DOutMax=[]  NOutMin=[]  NOutMax=[]  SumOutMin=[]  SumOutMax=[]  SaturationOutMin=[]  SaturationOutMax=[]  PParamMin=[]  PParamMax=[]  IParamMin=[]  IParamMax=[]  DParamMin=[]  DParamMax=[]  NParamMin=[]  NParamMax=[]  KbParamMin=[]  KbParamMax=[]  KtParamMin=[]  KtParamMax=[]  KbOutMin=[]  KbOutMax=[]  KtOutMin=[]  KtOutMax=[]  IntegratorOutMin=[]  IntegratorOutMax=[]  FilterOutMin=[]  FilterOutMax=[]  SumI1OutMin=[]  SumI1OutMax=[]  SumI2OutMin=[]  SumI2OutMax=[]  SumI3OutMin=[]  SumI3OutMax=[]  SumI4OutMin=[]  SumI4OutMax=[]  SumDOutMin=[]  SumDOutMax=[]  DifferentiatorOutMin=[]  DifferentiatorOutMax=[]  FilterDiffOutCoefMin=[]  FilterDiffOutCoefMax=[]  ReciprocalOutMin=[]  ReciprocalOutMax=[]  SumDenOutMin=[]  SumDenOutMax=[]  SumNumOutMin=[]  SumNumOutMax=[]  DivideOutMin=[]  DivideOutMax=[]  IntegratorContinuousStateAttributes=''  IntegratorStateMustResolveToSignalObject=off  IntegratorRTWStateStorageClass=Auto  FilterContinuousStateAttributes=''  FilterStateMustResolveToSignalObject=off  FilterRTWStateStorageClass=Auto  ParallelPVariant=InternalParameters  IdealPVariant=Disabled  IVariant=InternalParameters  DVariant=InternalParameters  IntegratorVariant=Discrete  SatVariant=Enabled  AWVariant=Passthrough  PCopyVariant=Disabled  TRVariant=Disabled  FdbkBlocksVariant=Forward  IdealPFdbkVariant=Disabled  SatFdbkVariant=Disabled  DerivativeFilterVariant=ForwardEulerFilter  NVariant=InternalParameters  NCopyVariant=Disabled  FilterICVariant=InternalICsFilter  IntegratorICVariant=InternalICs  ExternalResetVariant=Disabled  TRSumVariant=Passthrough  SumFdbkVariant=Disabled  SumVariant=Sum_PID
  Roll Controller : simulink/Continuous/PID Controller  Controller=PID  Form=Parallel  TimeDomain=Discrete-time  SampleTime=-1  IntegratorMethod=Forward Euler  FilterMethod=Forward Euler  ControllerParametersSource=internal  P=1  I=1  D=0  UseFilter=on  N=100  TunerSelectOption=Transfer Function Based (PID Tuner App)  InitialConditionSource=internal  InitialConditionForIntegrator=0  InitialConditionForFilter=0  DifferentiatorICPrevScaledInput=0  ExternalReset=none  TrackingMode=off  Kt=1  LimitOutput=on  UpperSaturationLimit=500  LowerSaturationLimit=-500  LinearizeAsGain=off  AntiWindupMode=clamping  Kb=1  RndMeth=Simplest  POutMin=[]  POutMax=[]  IOutMin=[]  IOutMax=[]  DOutMin=[]  DOutMax=[]  NOutMin=[]  NOutMax=[]  SumOutMin=[]  SumOutMax=[]  SaturationOutMin=[]  SaturationOutMax=[]  PParamMin=[]  PParamMax=[]  IParamMin=[]  IParamMax=[]  DParamMin=[]  DParamMax=[]  NParamMin=[]  NParamMax=[]  KbParamMin=[]  KbParamMax=[]  KtParamMin=[]  KtParamMax=[]  KbOutMin=[]  KbOutMax=[]  KtOutMin=[]  KtOutMax=[]  IntegratorOutMin=[]  IntegratorOutMax=[]  FilterOutMin=[]  FilterOutMax=[]  SumI1OutMin=[]  SumI1OutMax=[]  SumI2OutMin=[]  SumI2OutMax=[]  SumI3OutMin=[]  SumI3OutMax=[]  SumI4OutMin=[]  SumI4OutMax=[]  SumDOutMin=[]  SumDOutMax=[]  DifferentiatorOutMin=[]  DifferentiatorOutMax=[]  FilterDiffOutCoefMin=[]  FilterDiffOutCoefMax=[]  ReciprocalOutMin=[]  ReciprocalOutMax=[]  SumDenOutMin=[]  SumDenOutMax=[]  SumNumOutMin=[]  SumNumOutMax=[]  DivideOutMin=[]  DivideOutMax=[]  IntegratorContinuousStateAttributes=''  IntegratorStateMustResolveToSignalObject=off  IntegratorRTWStateStorageClass=Auto  FilterContinuousStateAttributes=''  FilterStateMustResolveToSignalObject=off  FilterRTWStateStorageClass=Auto  ParallelPVariant=InternalParameters  IdealPVariant=Disabled  IVariant=InternalParameters  DVariant=InternalParameters  IntegratorVariant=Discrete  SatVariant=Enabled  AWVariant=DiscClampingParallel  PCopyVariant=Disabled  TRVariant=Disabled  FdbkBlocksVariant=Forward  IdealPFdbkVariant=Disabled  SatFdbkVariant=Disabled  DerivativeFilterVariant=ForwardEulerFilter  NVariant=InternalParameters  NCopyVariant=Disabled  FilterICVariant=InternalICsFilter  IntegratorICVariant=InternalICs  ExternalResetVariant=Disabled  TRSumVariant=Passthrough  SumFdbkVariant=Disabled  SumVariant=Sum_PID
  Sum : Sum  Inputs=-+
  Sum1 : Sum  Inputs=+-
  Aileron : Outport
  wires:
  Current Roll Angle/1 -> Sum1/2
  Aileron Controller/1 -> Aileron/1
  Sum1/1 -> Aileron Controller/1
  Roll Controller/1 -> Sum1/1
  Sum/1 -> Roll Controller/1
  Current Heading/1 -> Sum/1
  Demanded Heading/1 -> Sum/2

== system Hardware_deploy_model/Sensors/Error State Kalman Filter/Wraparound Heading ==
  In1 : Inport
  Abs : Abs
  Constant : Constant  Value=360  OutDataTypeStr=single
  Demux : Demux  Outputs=3
  Mux : Mux  Inputs=3
  Subtract : Sum  Inputs=-+
  Switch : Switch  Criteria=u2 > Threshold  OutDataTypeStr=single
  Out1 : Outport
  wires:
  In1/1 -> Demux/1
  Mux/1 -> Out1/1
  Demux/1 -> Mux/1
  Demux/2 -> Mux/2
  Demux/3 -> Abs/1, Switch/2, Switch/1
  Switch/1 -> Mux/3
  Subtract/1 -> Switch/3
  Constant/1 -> Subtract/2
  Abs/1 -> Subtract/1

== system Hardware_deploy_model/Sensors/GPS Init/If Action Subsystem ==
  GPS_LL : Inport
  GPS_Alt : Inport  Port=2
  Action Port : ActionPort  ActionPortLabel=if(u1 & u2)
  Constant : Constant  Value=false
  Data Store Write : DataStoreWrite  DataStoreName=GPS_Init_LL
  Data Store Write1 : DataStoreWrite  DataStoreName=GPS_init
  Data Store Write2 : DataStoreWrite  DataStoreName=GPS_ref_height  DataStoreElements=GPS_ref_height
  wires:
  Constant/1 -> Data Store Write1/1
  GPS_LL/1 -> Data Store Write/1
  GPS_Alt/1 -> Data Store Write2/1

== system Hardware_deploy_model/Sensors/LLA to Flat Earth/LatLong wrap ==
  LatLong : Inport  OutDataTypeStr=single
  Constant : Constant  Value=180  OutDataTypeStr=single
  Constant1 : Constant  Value=0  OutDataTypeStr=single
  Demux : Demux  Outputs=2
  Latitude Wrap 90 : Subsystem  AncestorBlock=aerolibtransform2sys/Latitude Wrap 90  mask(LatitudeWrap90){}
      mask init:
      | aeroicon('aeroblk')
  Mux : Mux  Inputs=2
  Sum : Sum  Inputs=|++
  Switch1 : Switch  Criteria=u2 ~= 0  OutDataTypeStr=single
  Wrap Longitude : Subsystem  AncestorBlock=aerolibtransform2sys/Wrap Angle 180
      mask init:
      | aeroicon('aeroblk');
  Lat/Long wrapped : Outport  OutDataTypeStr=single
  wires:
  Latitude Wrap 90/1(Lat wrapped) -> Mux/1
  Latitude Wrap 90/2(Wrap flag) -> Switch1/2
  Demux/1 -> Latitude Wrap 90/1(Lat)
  Wrap Longitude/1(Angle 180) -> Mux/2
  Mux/1 -> Lat/Long wrapped/1
  Sum/1 -> Wrap Longitude/1(Angle)
  Demux/2 -> Sum/2
  Switch1/1 -> Sum/1
  Constant1/1 -> Switch1/3
  Constant/1 -> Switch1/1
  LatLong/1 -> Demux/1

== system Hardware_deploy_model/Sensors/LLA to Flat Earth/LatLong wrap LL0 ==
  LatLong : Inport
  Constant : Constant  Value=180  OutDataTypeStr=single
  Constant1 : Constant  Value=0  OutDataTypeStr=single
  Demux : Demux  Outputs=2
  Latitude Wrap 90 : Subsystem  AncestorBlock=aerolibtransform2sys/Latitude Wrap 90  mask(LatitudeWrap90){}
      mask init:
      | aeroicon('aeroblk')
  Mux : Mux  Inputs=2
  Sum : Sum  Inputs=|++
  Switch1 : Switch  Criteria=u2 ~= 0
  Wrap Longitude : Subsystem  AncestorBlock=aerolibtransform2sys/Wrap Angle 180
      mask init:
      | aeroicon('aeroblk');
  Lat/Long wrapped : Outport
  wires:
  Latitude Wrap 90/1(Lat wrapped) -> Mux/1
  Latitude Wrap 90/2(Wrap flag) -> Switch1/2
  Demux/1 -> Latitude Wrap 90/1(Lat)
  Wrap Longitude/1(Angle 180) -> Mux/2
  Mux/1 -> Lat/Long wrapped/1
  Sum/1 -> Wrap Longitude/1(Angle)
  Demux/2 -> Sum/2
  Switch1/1 -> Sum/1
  Constant1/1 -> Switch1/3
  Constant/1 -> Switch1/1
  LatLong/1 -> Demux/1

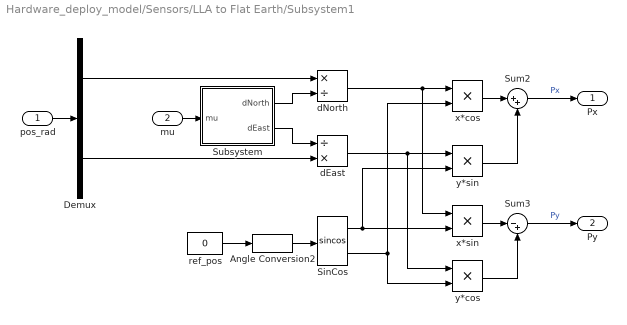
== system Hardware_deploy_model/Sensors/LLA to Flat Earth/Subsystem1 ==
  pos_rad : Inport
  mu : Inport  Port=2
  Angle Conversion2 : aerolibtransform2/LLA to Flat Earth/Subsystem/Angle Conversion2  SystemSampleTime=-1
      settings: SourceProductName=Aerospace Blockset  SourceProductBaseCode=AE
  Demux : Demux  Outputs=2
  SinCos : Trigonometry  Operator=sincos
  Subsystem : Subsystem
  Sum2 : Sum  Inputs=|++
  Sum3 : Sum  Inputs=|-+
  dEast : Product  Inputs=/*  RndMeth=Zero
  dNorth : Product  Inputs=*/  RndMeth=Zero
  ref_pos : Constant  Value=0  OutDataTypeStr=single
  x*cos : Product  RndMeth=Zero
  x*sin : Product  RndMeth=Zero
  y*cos : Product  RndMeth=Zero
  y*sin : Product  RndMeth=Zero
  Px : Outport
  Py : Outport  Port=2
  wires:
  x*cos/1 -> Sum2/1
  pos_rad/1 -> Demux/1
  SinCos/1 -> y*sin/2, x*sin/2
  mu/1 -> Subsystem/1(mu)
  Sum2/1 -> Px/1  "Px"
  x*sin/1 -> Sum3/1
  y*sin/1 -> Sum2/2
  SinCos/2 -> x*cos/2, y*cos/2
  y*cos/1 -> Sum3/2
  Demux/2 -> dEast/2
  Subsystem/1(dNorth) -> dNorth/2
  Subsystem/2(dEast) -> dEast/1
  Demux/1 -> dNorth/1
  dEast/1 -> y*sin/1, y*cos/1
  ref_pos/1 -> Angle Conversion2/1
  dNorth/1 -> x*cos/1, x*sin/1
  Angle Conversion2/1 -> SinCos/1
  Sum3/1 -> Py/1  "Py"

== system Hardware_deploy_model/GNC/HDG_ALT Hold/Altitude Hold/Altitude Hold ==
  In1 : Inport
  In2 : Inport  Port=2
  theta : Inport  Port=3
  Elevator Controller : simulink/Continuous/PID Controller  Controller=PID  Form=Parallel  TimeDomain=Discrete-time  SampleTime=-1  IntegratorMethod=Forward Euler  FilterMethod=Forward Euler  ControllerParametersSource=internal  P=1  I=1  D=0  UseFilter=on  N=100  TunerSelectOption=Transfer Function Based (PID Tuner App)  InitialConditionSource=internal  InitialConditionForIntegrator=0  InitialConditionForFilter=0  DifferentiatorICPrevScaledInput=0  ExternalReset=none  TrackingMode=off  Kt=1  LimitOutput=on  UpperSaturationLimit=500  LowerSaturationLimit=-500  LinearizeAsGain=off  AntiWindupMode=none  Kb=1  RndMeth=Simplest  POutMin=[]  POutMax=[]  IOutMin=[]  IOutMax=[]  DOutMin=[]  DOutMax=[]  NOutMin=[]  NOutMax=[]  SumOutMin=[]  SumOutMax=[]  SaturationOutMin=[]  SaturationOutMax=[]  PParamMin=[]  PParamMax=[]  IParamMin=[]  IParamMax=[]  DParamMin=[]  DParamMax=[]  NParamMin=[]  NParamMax=[]  KbParamMin=[]  KbParamMax=[]  KtParamMin=[]  KtParamMax=[]  KbOutMin=[]  KbOutMax=[]  KtOutMin=[]  KtOutMax=[]  IntegratorOutMin=[]  IntegratorOutMax=[]  FilterOutMin=[]  FilterOutMax=[]  SumI1OutMin=[]  SumI1OutMax=[]  SumI2OutMin=[]  SumI2OutMax=[]  SumI3OutMin=[]  SumI3OutMax=[]  SumI4OutMin=[]  SumI4OutMax=[]  SumDOutMin=[]  SumDOutMax=[]  DifferentiatorOutMin=[]  DifferentiatorOutMax=[]  FilterDiffOutCoefMin=[]  FilterDiffOutCoefMax=[]  ReciprocalOutMin=[]  ReciprocalOutMax=[]  SumDenOutMin=[]  SumDenOutMax=[]  SumNumOutMin=[]  SumNumOutMax=[]  DivideOutMin=[]  DivideOutMax=[]  IntegratorContinuousStateAttributes=''  IntegratorStateMustResolveToSignalObject=off  IntegratorRTWStateStorageClass=Auto  FilterContinuousStateAttributes=''  FilterStateMustResolveToSignalObject=off  FilterRTWStateStorageClass=Auto  ParallelPVariant=InternalParameters  IdealPVariant=Disabled  IVariant=InternalParameters  DVariant=InternalParameters  IntegratorVariant=Discrete  SatVariant=Enabled  AWVariant=Passthrough  PCopyVariant=Disabled  TRVariant=Disabled  FdbkBlocksVariant=Forward  IdealPFdbkVariant=Disabled  SatFdbkVariant=Disabled  DerivativeFilterVariant=ForwardEulerFilter  NVariant=InternalParameters  NCopyVariant=Disabled  FilterICVariant=InternalICsFilter  IntegratorICVariant=InternalICs  ExternalResetVariant=Disabled  TRSumVariant=Passthrough  SumFdbkVariant=Disabled  SumVariant=Sum_PID
  Pitch Controller : simulink/Continuous/PID Controller  Controller=PID  Form=Parallel  TimeDomain=Discrete-time  SampleTime=-1  IntegratorMethod=Forward Euler  FilterMethod=Forward Euler  ControllerParametersSource=internal  P=1  I=1  D=0  UseFilter=on  N=100  TunerSelectOption=Transfer Function Based (PID Tuner App)  InitialConditionSource=internal  InitialConditionForIntegrator=0  InitialConditionForFilter=0  DifferentiatorICPrevScaledInput=0  ExternalReset=none  TrackingMode=off  Kt=1  LimitOutput=on  UpperSaturationLimit=500  LowerSaturationLimit=-500  LinearizeAsGain=off  AntiWindupMode=none  Kb=1  RndMeth=Simplest  POutMin=[]  POutMax=[]  IOutMin=[]  IOutMax=[]  DOutMin=[]  DOutMax=[]  NOutMin=[]  NOutMax=[]  SumOutMin=[]  SumOutMax=[]  SaturationOutMin=[]  SaturationOutMax=[]  PParamMin=[]  PParamMax=[]  IParamMin=[]  IParamMax=[]  DParamMin=[]  DParamMax=[]  NParamMin=[]  NParamMax=[]  KbParamMin=[]  KbParamMax=[]  KtParamMin=[]  KtParamMax=[]  KbOutMin=[]  KbOutMax=[]  KtOutMin=[]  KtOutMax=[]  IntegratorOutMin=[]  IntegratorOutMax=[]  FilterOutMin=[]  FilterOutMax=[]  SumI1OutMin=[]  SumI1OutMax=[]  SumI2OutMin=[]  SumI2OutMax=[]  SumI3OutMin=[]  SumI3OutMax=[]  SumI4OutMin=[]  SumI4OutMax=[]  SumDOutMin=[]  SumDOutMax=[]  DifferentiatorOutMin=[]  DifferentiatorOutMax=[]  FilterDiffOutCoefMin=[]  FilterDiffOutCoefMax=[]  ReciprocalOutMin=[]  ReciprocalOutMax=[]  SumDenOutMin=[]  SumDenOutMax=[]  SumNumOutMin=[]  SumNumOutMax=[]  DivideOutMin=[]  DivideOutMax=[]  IntegratorContinuousStateAttributes=''  IntegratorStateMustResolveToSignalObject=off  IntegratorRTWStateStorageClass=Auto  FilterContinuousStateAttributes=''  FilterStateMustResolveToSignalObject=off  FilterRTWStateStorageClass=Auto  ParallelPVariant=InternalParameters  IdealPVariant=Disabled  IVariant=InternalParameters  DVariant=InternalParameters  IntegratorVariant=Discrete  SatVariant=Enabled  AWVariant=Passthrough  PCopyVariant=Disabled  TRVariant=Disabled  FdbkBlocksVariant=Forward  IdealPFdbkVariant=Disabled  SatFdbkVariant=Disabled  DerivativeFilterVariant=ForwardEulerFilter  NVariant=InternalParameters  NCopyVariant=Disabled  FilterICVariant=InternalICsFilter  IntegratorICVariant=InternalICs  ExternalResetVariant=Disabled  TRSumVariant=Passthrough  SumFdbkVariant=Disabled  SumVariant=Sum_PID
  Sum : Sum  Inputs=+-
  Sum1 : Sum  Inputs=+-
  Elevator : Outport
  wires:
  Pitch Controller/1 -> Sum1/1
  theta/1 -> Sum1/2
  In2/1 -> Sum/2
  Sum/1 -> Pitch Controller/1
  Elevator Controller/1 -> Elevator/1  "Elevator"
  In1/1 -> Sum/1
  Sum1/1 -> Elevator Controller/1

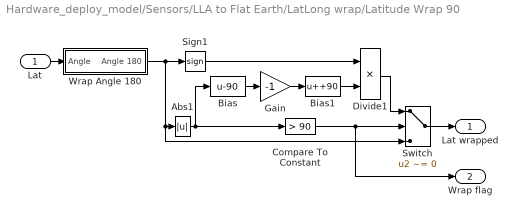
== system Hardware_deploy_model/Sensors/LLA to Flat Earth/LatLong wrap/Latitude Wrap 90 ==
  Lat : Inport
  Abs1 : Abs
  Bias : Bias  Bias=-90
  Bias1 : Bias  Bias=+90
  Compare To Constant : simulink/Logic and Bit Operations/Compare To Constant  relop=>  const=90  OutDataTypeStr=boolean
  Divide1 : Product  Inputs=**
  Gain : Gain  Gain=-1
  Sign1 : Signum
  Switch : Switch  Criteria=u2 ~= 0  OutDataTypeStr=single
  Wrap Angle 180 : Subsystem  AncestorBlock=aerolibtransform2sys/Wrap Angle 180
      mask init:
      | aeroicon('aeroblk');
  Lat wrapped : Outport
  Wrap flag : Outport  Port=2
  wires:
  Compare To Constant/1 -> Switch/2, Wrap flag/1
  Wrap Angle 180/1(Angle 180) -> Sign1/1, Switch/3, Abs1/1
  Lat/1 -> Wrap Angle 180/1(Angle)
  Abs1/1 -> Compare To Constant/1, Bias/1
  Bias/1 -> Gain/1
  Gain/1 -> Bias1/1
  Bias1/1 -> Divide1/2
  Sign1/1 -> Divide1/1
  Divide1/1 -> Switch/1
  Switch/1 -> Lat wrapped/1

== system Hardware_deploy_model/Sensors/LLA to Flat Earth/LatLong wrap/Wrap Longitude ==
  Angle : Inport
  Abs : Abs
  Bias : Bias  Bias=180
  Bias1 : Bias  Bias=-180
  Compare To Constant : simulink/Logic and Bit Operations/Compare To Constant  relop=>  const=180  OutDataTypeStr=boolean
  Constant2 : Constant  Value=360  OutDataTypeStr=single
  Math Function1 : Math  Operator=mod  SaturateOnIntegerOverflow=on
  Switch : Switch  Criteria=u2 ~= 0  Threshold=180
  Angle 180 : Outport
  wires:
  Compare To Constant/1 -> Switch/2
  Angle/1 -> Bias/1, Switch/3, Abs/1
  Abs/1 -> Compare To Constant/1
  Bias/1 -> Math Function1/1
  Constant2/1 -> Math Function1/2
  Math Function1/1 -> Bias1/1
  Bias1/1 -> Switch/1
  Switch/1 -> Angle 180/1

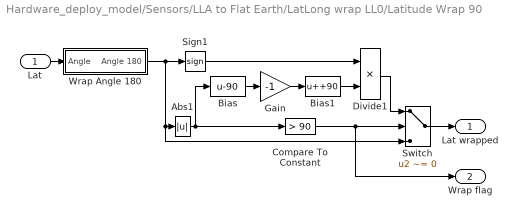
== system Hardware_deploy_model/Sensors/LLA to Flat Earth/LatLong wrap LL0/Latitude Wrap 90 ==
  Lat : Inport
  Abs1 : Abs
  Bias : Bias  Bias=-90
  Bias1 : Bias  Bias=+90
  Compare To Constant : simulink/Logic and Bit Operations/Compare To Constant  relop=>  const=90  OutDataTypeStr=boolean
  Divide1 : Product  Inputs=**
  Gain : Gain  Gain=-1
  Sign1 : Signum
  Switch : Switch  Criteria=u2 ~= 0
  Wrap Angle 180 : Subsystem  AncestorBlock=aerolibtransform2sys/Wrap Angle 180
      mask init:
      | aeroicon('aeroblk');
  Lat wrapped : Outport
  Wrap flag : Outport  Port=2
  wires:
  Compare To Constant/1 -> Switch/2, Wrap flag/1
  Wrap Angle 180/1(Angle 180) -> Sign1/1, Switch/3, Abs1/1
  Lat/1 -> Wrap Angle 180/1(Angle)
  Abs1/1 -> Compare To Constant/1, Bias/1
  Bias/1 -> Gain/1
  Gain/1 -> Bias1/1
  Bias1/1 -> Divide1/2
  Sign1/1 -> Divide1/1
  Divide1/1 -> Switch/1
  Switch/1 -> Lat wrapped/1

== system Hardware_deploy_model/Sensors/LLA to Flat Earth/LatLong wrap LL0/Wrap Longitude ==
  Angle : Inport
  Abs : Abs
  Bias : Bias  Bias=180
  Bias1 : Bias  Bias=-180
  Compare To Constant : simulink/Logic and Bit Operations/Compare To Constant  relop=>  const=180  OutDataTypeStr=boolean
  Constant2 : Constant  Value=360  OutDataTypeStr=single
  Math Function1 : Math  Operator=mod  SaturateOnIntegerOverflow=on
  Switch : Switch  Criteria=u2 ~= 0  Threshold=180
  Angle 180 : Outport
  wires:
  Compare To Constant/1 -> Switch/2
  Angle/1 -> Bias/1, Switch/3, Abs/1
  Abs/1 -> Compare To Constant/1
  Bias/1 -> Math Function1/1
  Constant2/1 -> Math Function1/2
  Math Function1/1 -> Bias1/1
  Bias1/1 -> Switch/1
  Switch/1 -> Angle 180/1

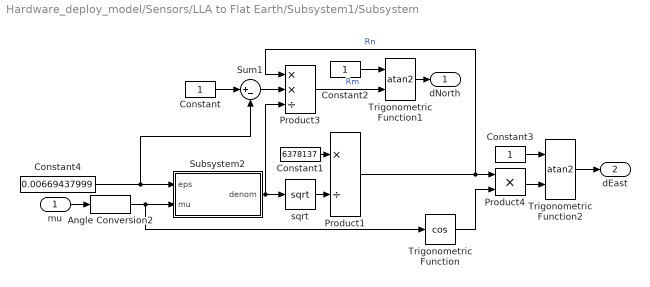
== system Hardware_deploy_model/Sensors/LLA to Flat Earth/Subsystem1/Subsystem ==
  mu : Inport
  Angle Conversion2 : aerolibtransform2/LLA to Flat Earth/Subsystem/Find Radian//Distance/Angle Conversion2  SystemSampleTime=-1
      settings: SourceProductName=Aerospace Blockset  SourceProductBaseCode=AE
  Constant : Constant  OutDataTypeStr=single
  Constant1 : Constant  Value=6378137  OutDataTypeStr=single
  Constant2 : Constant  OutDataTypeStr=single
  Constant3 : Constant  OutDataTypeStr=single
  Constant4 : Constant  Value=0.00669437999  OutDataTypeStr=single
  Product1 : Product  Inputs=*/  RndMeth=Zero
  Product3 : Product  Inputs=**/  OutDataTypeStr=single  RndMeth=Zero
  Product4 : Product  RndMeth=Zero
  Subsystem2 : Subsystem
  Sum1 : Sum  Inputs=|+-
  Trigonometric Function : Trigonometry  Operator=cos
  Trigonometric Function1 : Trigonometry  Operator=atan2
  Trigonometric Function2 : Trigonometry  Operator=atan2
  sqrt : Sqrt  AlgorithmType=Newton-Raphson  SaturateOnIntegerOverflow=on
  dNorth : Outport
  dEast : Outport  Port=2
  wires:
  Angle Conversion2/1 -> Subsystem2/2(mu), Trigonometric Function/1
  Constant/1 -> Sum1/1
  Trigonometric Function2/1 -> dEast/1
  Constant2/1 -> Trigonometric Function1/1
  Constant4/1 -> Sum1/2, Subsystem2/1(eps)
  sqrt/1 -> Product1/2
  Subsystem2/1(denom) -> Product3/3, sqrt/1
  Trigonometric Function/1 -> Product4/2
  Product1/1 -> Product3/1, Product4/1  "Rn"
  Trigonometric Function1/1 -> dNorth/1
  Product3/1 -> Trigonometric Function1/2  "Rm"
  Sum1/1 -> Product3/2
  Product4/1 -> Trigonometric Function2/2
  Constant1/1 -> Product1/1
  Constant3/1 -> Trigonometric Function2/1
  mu/1 -> Angle Conversion2/1

== system Hardware_deploy_model/Sensors/LLA to Flat Earth/LatLong wrap/Latitude Wrap 90/Wrap Angle 180 ==
  Angle : Inport
  Abs : Abs
  Bias : Bias  Bias=180
  Bias1 : Bias  Bias=-180
  Compare To Constant : simulink/Logic and Bit Operations/Compare To Constant  relop=>  const=180  OutDataTypeStr=boolean
  Constant2 : Constant  Value=360  OutDataTypeStr=single
  Math Function1 : Math  Operator=mod  SaturateOnIntegerOverflow=on
  Switch : Switch  Criteria=u2 ~= 0  Threshold=180
  Angle 180 : Outport
  wires:
  Compare To Constant/1 -> Switch/2
  Angle/1 -> Bias/1, Switch/3, Abs/1
  Abs/1 -> Compare To Constant/1
  Bias/1 -> Math Function1/1
  Constant2/1 -> Math Function1/2
  Math Function1/1 -> Bias1/1
  Bias1/1 -> Switch/1
  Switch/1 -> Angle 180/1

== system Hardware_deploy_model/Sensors/LLA to Flat Earth/LatLong wrap LL0/Latitude Wrap 90/Wrap Angle 180 ==
  Angle : Inport
  Abs : Abs
  Bias : Bias  Bias=180
  Bias1 : Bias  Bias=-180
  Compare To Constant : simulink/Logic and Bit Operations/Compare To Constant  relop=>  const=180  OutDataTypeStr=boolean
  Constant : Constant  Value=360  OutDataTypeStr=single
  Math Function1 : Math  Operator=mod  SaturateOnIntegerOverflow=on
  Switch : Switch  Criteria=u2 ~= 0  Threshold=180
  Angle 180 : Outport
  wires:
  Compare To Constant/1 -> Switch/2
  Angle/1 -> Bias/1, Switch/3, Abs/1
  Abs/1 -> Compare To Constant/1
  Bias/1 -> Math Function1/1
  Constant/1 -> Math Function1/2
  Math Function1/1 -> Bias1/1
  Bias1/1 -> Switch/1
  Switch/1 -> Angle 180/1

== system Hardware_deploy_model/Sensors/LLA to Flat Earth/Subsystem1/Subsystem/Subsystem2 ==
  eps : Inport
  mu : Inport  Port=2
  Constant : Constant  OutDataTypeStr=single
  Product1 : Product  Inputs=3  OutDataTypeStr=single  RndMeth=Zero
  Sum1 : Sum  Inputs=|+-
  Trigonometric Function1 : Trigonometry
  denom : Outport
  wires:
  Product1/1 -> Sum1/2
  Trigonometric Function1/1 -> Product1/2, Product1/3
  Constant/1 -> Sum1/1
  eps/1 -> Product1/1
  Sum1/1 -> denom/1
  mu/1 -> Trigonometric Function1/1
